simulink model "led_on"  (R2023b)
settings: Solver=FixedStepDiscrete  StartTime=0.0  StopTime=inf  FixedStep=1  RelTol=1e-3
settings Model: Creator=Beshary  LastModifiedBy=Beshary

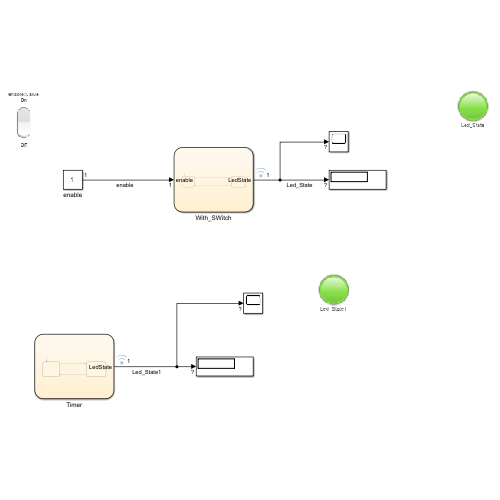
[thumbnail: Simulink's stored preview of the top-level diagram]
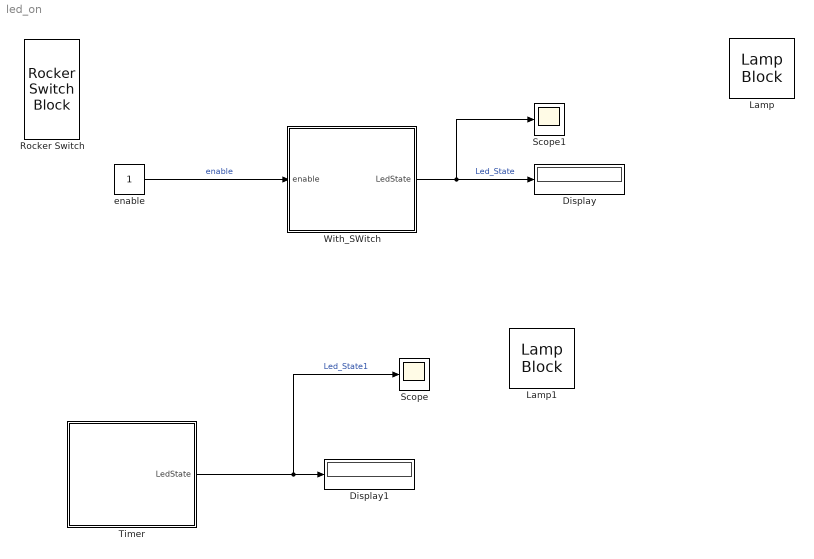
== system led_on ==
  Display : Display
  Display1 : Display
  Lamp : LampBlock  LabelPosition=Bottom
  Lamp1 : LampBlock  LabelPosition=Bottom
  Rocker Switch : RockerSwitchBlock
      settings: Values={{'Off', 'On'}, [0 1]}
  Scope : Scope
  Scope1 : Scope
  Timer : Stateflow chart  TreatAsAtomicUnit=on
  With_SWitch : Stateflow chart  TreatAsAtomicUnit=on
  enable : Constant
  wires:
  enable/1 -> With_SWitch/1(enable)  "enable"
  With_SWitch/1(LedState) -> Scope1/1, Display/1  "Led_State"
  Timer/1(LedState) -> Scope/1, Display1/1  "Led_State1"

== stateflow chart led_on/Timer ==
  state LedOff
    en:
    LedState=0;
  state LedOn
    en:
    LedState=1;
  (default) -> LedOff
  LedOff -> LedOn : after(1,sec)
  LedOn -> LedOff : after(1,sec)
  data: LedState output

== stateflow chart led_on/With_SWitch ==
  state LedOff
    en:
    LedState=0;
  state LedOn
    en:
    LedState=1;
  (default) -> LedOff
  LedOff -> LedOn : [enable==1]{after(1,sec)}
  LedOn -> LedOff : after(1,sec)
  data: enable input; LedState output
